simulink model "sfserratura"  (Simulink 7.2)
settings: Solver=FixedStepDiscrete  StartTime=0.0  StopTime=inf  FixedStep=1  RelTol=1e-3
settings Model: Creator=gle  LastModifiedBy=gle  ExtModeTrigMode=oneshot  ExtModeArmWhenConnect=off
settings DataIOCC: LimitDataPoints=off  SignalLoggingName=sigsOut
settings OptimizationCC: BooleanDataType=off
settings DebuggingCC: SaveWithParameterizedLinksMsg=none  SignalResolutionControl=TryResolveAllWithWarning  SolverPrmCheckMsg=none  MultiTaskDSMMsg=warning  MultiTaskCondExecSysMsg=none  StrictBusMsg=None
settings HardwareCC: TargetUnknown=on
settings RTWCC: IncludeERTFirstTime=on

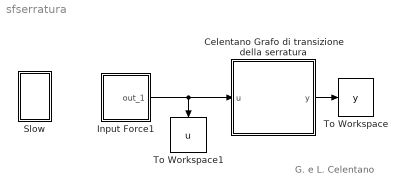
== system sfserratura ==
  note: G. e L. Celentano
  Celentano Grafo di transizione della serratura : Stateflow chart
  Input Force1 : Subsystem  mask(Repeating table){rep_seq_t=[0 :4], rep_seq_y=[1 3 4 3 1 ]}
      mask prompts: rep_seq_t "Time values:"; rep_seq_y "Output values:"
      mask help: Repeating table.
      mask init:
      | period = max(rep_seq_t);
      mask Help: Repeats cycle given in table. Time values should be monotonically increasing.
      mask Display: plot([rep_seq_t,rep_seq_t+period,rep_seq_t+2*period,rep_seq_t(1)+3*period],[rep_seq_y,rep_seq_y,rep_seq_y,rep_seq_y(1)])
  Slow : Subsystem
      mask Display: plot([0 1],[0 1])
  To Workspace : ToWorkspace  VariableName=y  SampleTime=-1  SaveFormat=Array
  To Workspace1 : ToWorkspace  VariableName=u  SampleTime=-1  SaveFormat=Array
      settings: Orientation=down
  wires:
  Celentano Grafo di transizione della serratura/1(y) -> To Workspace/1
  Input Force1/1(out_1) -> Celentano Grafo di transizione della serratura/1(u), To Workspace1/1

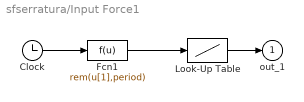
== system sfserratura/Input Force1 ==
  Clock : Clock
      settings: Decimation=10
  Fcn1 : Fcn  Expr=rem(u[1],period)
  Look-Up Table : Lookup  InputValues=rep_seq_t  Table=rep_seq_y  OutDataType=sfix(16)  OutScaling=2^0  SaturateOnIntegerOverflow=on
  out_1 : Outport  InitialOutput=0
  wires:
  Look-Up Table/1 -> out_1/1
  Clock/1 -> Fcn1/1
  Fcn1/1 -> Look-Up Table/1

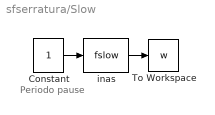
== system sfserratura/Slow ==
  note: Periodo
      | pause
  Constant : Constant  OutDataType=sfix(16)  OutScaling=2^0
  To Workspace : ToWorkspace  VariableName=w  SampleTime=-1  SaveFormat=Array
  inas : MATLABFcn  MATLABFcn=fslow
  wires:
  Constant/1 -> inas/1
  inas/1 -> To Workspace/1

== stateflow chart Celentano Grafo di transizione della serratura ==
  state x1/
    y=0;
  state x2/
    y=0;
  state x5/
    y=1;
  state x3/
    y=0;
  state x4/
    y=0;
  x1 -> x1 [order 1] : [u==1|u==2|u==4]
  x2 -> x2 [order 1] : [u==3]
  x1 -> x2 [order 2] : [u==3]
  (default) -> x1
  x2 -> x1 [order 3] : [u==1|u==2]
  x5 -> x2 [order 2] : [u==3]
  x5 -> x1 [order 1] : [u==1|u==2|u==4]
  x4 -> x2 [order 2] : [u==3]
  x2 -> x3 [order 2] : [u==4]
  x4 -> x5 [order 1] : [u==1]
  x4 -> x3 [order 3] : [u==4]
  x3 -> x4 : [u==3]
  data: u input double; y output double
